simulink model "AESEncryption_21821"  (R2018b)
settings: Solver=FixedStepDiscrete  StartTime=0.0  StopTime=10  RelTol=1e-3
undefined symbols (not defined in the file or in its folder): gray
libraries: hdlsllib x5, visionsources x1, dspmtrx3 x1
settings Model: Creator=Administrator  LastModifiedBy=Administrator
settings OptimizationCC: BlockReduction=off  ConditionallyExecuteInputs=off  DefaultParameterBehavior=Inlined
settings DebuggingCC: AlgebraicLoopMsg=error  SingleTaskRateTransMsg=error
settings HardwareCC: ProdBitPerPointer=32  ProdBitPerSizeT=32  ProdBitPerPtrDiffT=32  ProdLargestAtomicFloat=None  ProdIntDivRoundTo=Undefined  ProdEndianess=Unspecified  ProdWordSize=32  ProdHWDeviceType=ASIC/FPGA->ASIC/FPGA  TargetBitPerPointer=64  TargetBitPerSizeT=64  TargetBitPerPtrDiffT=64  TargetLongLongMode=on  TargetIntDivRoundTo=Zero  TargetEndianess=LittleEndian  TargetWordSize=64  TargetHWDeviceType=Custom Processor->MATLAB Host Computer  ProdEqTarget=off

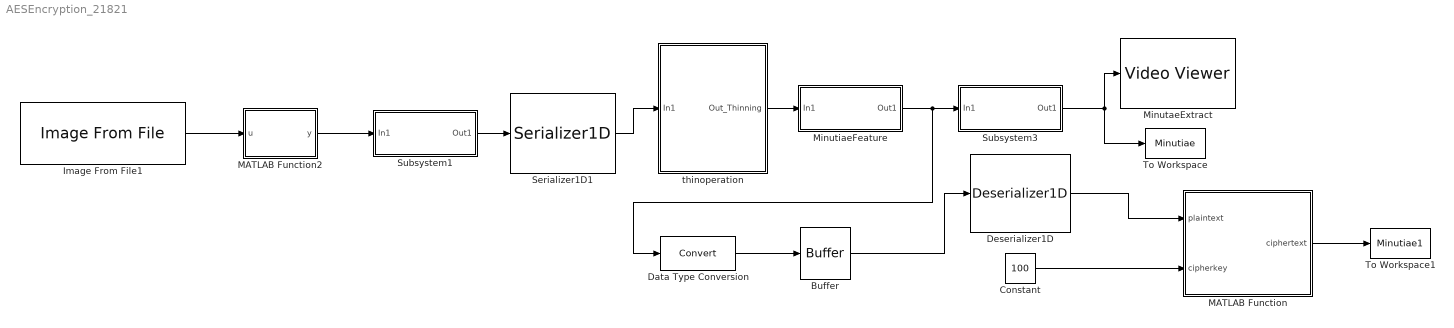
== system AESEncryption_21821 ==
  Buffer : Buffer  N=8192  OutputFrames=off
  Constant : Constant  Value=100  OutDataTypeStr=double
  Data Type Conversion : DataTypeConversion
  Deserializer1D : hdlsllib/HDL Operations/Deserializer1D  Ratio=128  IdleCycles=0  InitialCondition=0  startIn=off  validIn=off  validOut=off  inputDataDimensions=-1  inputSampleTime=-1  inputSignalType=auto
      settings: SourceProductName=HDL Coder  SourceProductBaseCode=HD
  Image From File1 : visionsources/Image From File  Tag=vipblks_nd  FileName=C:\Users\Administrator\Desktop\chapter\101_4.tif  imagePorts=One multidimensional signal  Ts=0.1  ImageDataType=uint8  Signed=on  WordLength=16  sdImageDataType=uint(8)  FractionLengthMode=User-defined  FractionLength=15  OutPortLabels=R|G|B
      settings: SourceProductName=Computer Vision System Toolbox
  MATLAB Function : MATLAB Function  TreatAsAtomicUnit=on
  MATLAB Function2 : MATLAB Function  TreatAsAtomicUnit=on
  MinutaeExtract : VideoViewer  colormapValue=gray(256)  FigPos=[367 903 376 593]
  MinutiaeFeature : Subsystem  TreatAsAtomicUnit=on
  Serializer1D1 : hdlsllib/HDL Operations/Serializer1D  Ratio=1  IdleCycles=0  validIn=off  startOut=off  validOut=off  inputDataDimensions=8192  inputSampleTime=-1  inputSignalType=auto
      settings: SourceProductName=HDL Coder  SourceProductBaseCode=HD
  Subsystem1 : Subsystem
  Subsystem3 : Subsystem
  To Workspace : ToWorkspace  VariableName=Minutiae  SampleTime=-1
      settings: Save2DSignal=2-D array (concatenate along first dimension)
  To Workspace1 : ToWorkspace  VariableName=Minutiae1  SampleTime=-1
      settings: Save2DSignal=2-D array (concatenate along first dimension)
  thinoperation : Subsystem  TreatAsAtomicUnit=on
  wires:
  Serializer1D1/1 -> thinoperation/1(In1)
  MATLAB Function2/1(y) -> Subsystem1/1(In1)
  Image From File1/1 -> MATLAB Function2/1(u)
  Subsystem1/1(Out1) -> Serializer1D1/1
  thinoperation/1(Out_Thinning) -> MinutiaeFeature/1(In1)
  Subsystem3/1(Out1) -> MinutaeExtract/1, To Workspace/1
  MATLAB Function/1(ciphertext) -> To Workspace1/1
  Constant/1 -> MATLAB Function/2(cipherkey)
  Deserializer1D/1 -> MATLAB Function/1(plaintext)
  MinutiaeFeature/1(Out1) -> Data Type Conversion/1, Subsystem3/1(In1)
  Data Type Conversion/1 -> Buffer/1
  Buffer/1 -> Deserializer1D/1

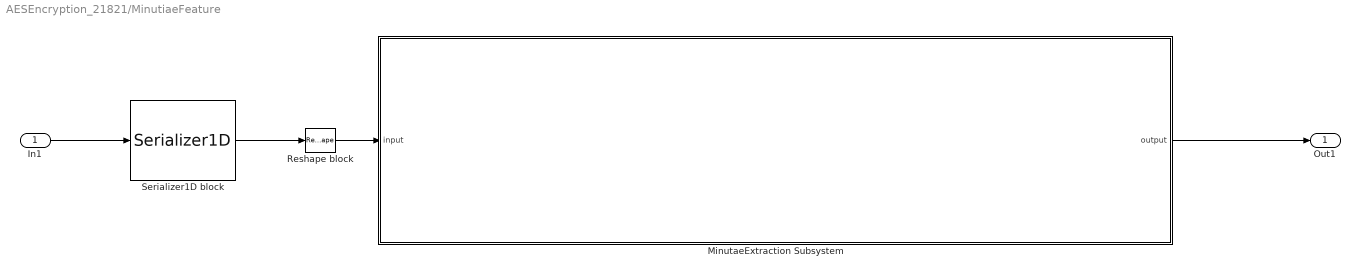
== system AESEncryption_21821/MinutiaeFeature ==
  In1 : Inport
  MinutaeExtraction Subsystem : Subsystem  TreatAsAtomicUnit=on
  Reshape block : Reshape  OutputDimensionality=Customize  OutputDimensions=[128,64]
  Serializer1D block : hdlsllib/HDL Operations/Serializer1D  Ratio=1  IdleCycles=0  validIn=off  startOut=off  validOut=off  inputDataDimensions=8192  inputSampleTime=-1  inputSignalType=auto
      settings: SourceProductName=HDL Coder  SourceProductBaseCode=HD
  Out1 : Outport
  wires:
  In1/1 -> Serializer1D block/1
  MinutaeExtraction Subsystem/1(output) -> Out1/1
  Reshape block/1 -> MinutaeExtraction Subsystem/1(input)
  Serializer1D block/1 -> Reshape block/1

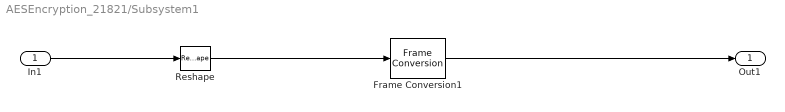
== system AESEncryption_21821/Subsystem1 ==
  In1 : Inport
  Frame Conversion1 : FrameConversion  OutFrame=Sample-based
  Reshape : Reshape
  Out1 : Outport
  wires:
  Frame Conversion1/1 -> Out1/1
  Reshape/1 -> Frame Conversion1/1
  In1/1 -> Reshape/1

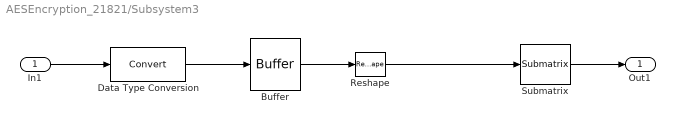
== system AESEncryption_21821/Subsystem3 ==
  In1 : Inport
  Buffer : Buffer  N=8192  OutputFrames=off
  Data Type Conversion : DataTypeConversion
  Reshape : Reshape  OutputDimensionality=Customize  OutputDimensions=[128,64]
  Submatrix : dspmtrx3/Submatrix  RowSpan=Range of rows  RowStartMode=First  RowStartIndex=1  RowEndMode=Last  RowEndIndex=1  ColSpan=Range of columns  ColStartMode=First  ColStartIndex=1  ColEndMode=Last  ColEndIndex=1
  Out1 : Outport
  wires:
  Data Type Conversion/1 -> Buffer/1
  Buffer/1 -> Reshape/1
  Reshape/1 -> Submatrix/1
  Submatrix/1 -> Out1/1
  In1/1 -> Data Type Conversion/1

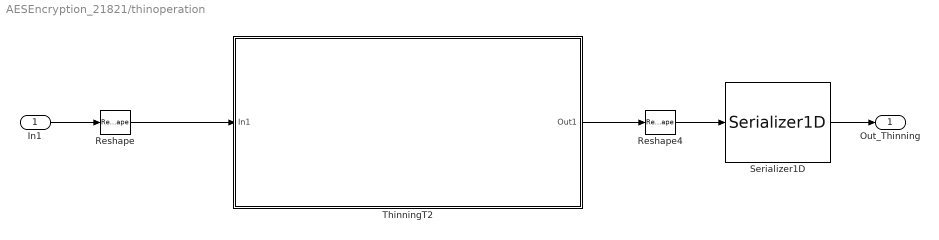
== system AESEncryption_21821/thinoperation ==
  In1 : Inport
  Reshape : Reshape  OutputDimensionality=Customize  OutputDimensions=[128,64]
  Reshape4 : Reshape  OutputDimensionality=Column vector (2-D)  OutputDimensions=[128,64]
  Serializer1D : hdlsllib/HDL Operations/Serializer1D  Ratio=1  IdleCycles=0  validIn=off  startOut=off  validOut=off  inputDataDimensions=-1  inputSampleTime=-1  inputSignalType=auto
      settings: SourceProductName=HDL Coder  SourceProductBaseCode=HD
  ThinningT2 : Subsystem  TreatAsAtomicUnit=on
  Out_Thinning : Outport
  wires:
  ThinningT2/1(Out1) -> Reshape4/1
  Reshape/1 -> ThinningT2/1(In1)
  Serializer1D/1 -> Out_Thinning/1
  In1/1 -> Reshape/1
  Reshape4/1 -> Serializer1D/1

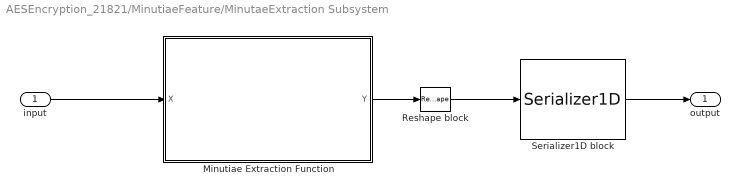
== system AESEncryption_21821/MinutiaeFeature/MinutaeExtraction Subsystem ==
  input : Inport
  Minutiae Extraction Function : MATLAB Function  TreatAsAtomicUnit=on
  Reshape block : Reshape  OutputDimensionality=Column vector (2-D)  OutputDimensions=[128,64]
  Serializer1D block : hdlsllib/HDL Operations/Serializer1D  Ratio=8192  IdleCycles=0  validIn=off  startOut=off  validOut=off  inputDataDimensions=-1  inputSampleTime=-1  inputSignalType=auto
      settings: SourceProductName=HDL Coder  SourceProductBaseCode=HD
  output : Outport
  wires:
  input/1 -> Minutiae Extraction Function/1(X)
  Serializer1D block/1 -> output/1
  Minutiae Extraction Function/1(Y) -> Reshape block/1
  Reshape block/1 -> Serializer1D block/1

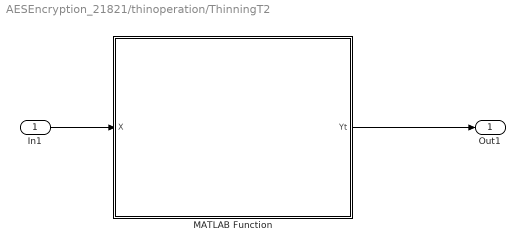
== system AESEncryption_21821/thinoperation/ThinningT2 ==
  In1 : Inport
  MATLAB Function : MATLAB Function  TreatAsAtomicUnit=on
  Out1 : Outport
  wires:
  In1/1 -> MATLAB Function/1(X)
  MATLAB Function/1(Yt) -> Out1/1

== matlab function AESEncryption_21821/MATLAB Function2 ==
  data: u input; y output
function y = fcn(u)
%#codegen
%i = rgb2gray(u);
b = u(100:227,150:213);
y = imbinarize(b);
%y = y(100:227,150:213);
%y = imbinarize(r);

== matlab function AESEncryption_21821/thinoperation/ThinningT2/MATLAB Function ==
  data: X input; Yt output
function Yt=thinningTh(X)
%img = imread ('2_4.jpg'); 
%Xr = rgb2gray(img);
%%%X = imbinarize(Xr);
%X = X(1:128,1:64);
[M,N]=size(X);
Yt = false(M,N);
Y=false(M,N,20);
Z=false(M,N,20);
Y(:,:,1)=X;
Z(:,:,1)=X;
for k=2:20
    Y(:,:,k)=Y(:,:,k-1);
    for i=2:M-1
        for j=2:N-1
            y11=Y(i-1,j-1,k);
            y12=Y(i-1,j,k);
            y13=Y(i-1,j+1,k);
            y21=Y(i,j-1,k);
            y22=Y(i,j,k);
            y23=Y(i,j+1,k);
            y31=Y(i+1,j-1,k);
            y32=Y(i+1,j,k);
            y33=Y(i+1,j+1,k);
            if y22==0
                if y11==1&&y12==1&&y13==1&&y31==0&&y32==0&&y33==0
                    Y(i,j,k)=1;
                elseif y11==1&&y13==0&&y21==1&&y23==0&&y31==1&&y33==0
                    Y(i,j,k)=1;
                elseif y11==0&&y12==0&&y13==0&&y31==1&&y32==1&&y33==1
                    Y(i,j,k)=1;
                elseif y11==0&&y13==1&&y21==0&&y23==1&&y31==0&&y33==1
                    Y(i,j,k)=1;
                elseif y12==1&&y13==1&&y21==0&&y23==1&&y32==0
                    Y(i,j,k)=1;
                elseif y11==1&&y12==1&&y21==1&&y23==0&&y32==0
                    Y(i,j,k)=1;
                elseif y12==0&&y21==1&&y23==0&&y31==1&&y21==1
                    Y(i,j,k)=1;
                elseif y12==0&&y21==0&&y23==1&&y32==1&&y33==1
                    Y(i,j,k)=1;
                    %extra
                elseif y11==0&&y12==0&&y23==1&&y31==1&&y32==1&&y33==1
                    Y(i,j,k)=1;
                end
            else
            end
        end
    end
%    Y(:,:,k)= Y(:,:,k-1);
     if Y(:,:,k)==Y(:,:,k-1)
%         break;
     end
end
Yt=Y(:,:,k);
%figure;
%imshow(Y);

== matlab function AESEncryption_21821/MATLAB Function ==
  data: plaintext input; ciphertext output; cipherkey input
%%%%%%%%%%%%%%%%%%%%%%%%%%%%%%%%%%%%%%%%%%%%%%%%%%%%%%%%%%%%%%%%%%%%%%%%%%
% MATLAB design: Advanced Encryption System (AES-128)
% [1] Advanced Encryption Standard (AES) (FIPS PUB 197)
%
% Key Design pattern covered in this example: 
% (1) This example uses fixed point and integer operators. 
% (2) Bitwise Operator support
%
%
% Note: This design is already in fixed point and suitable for HDL code
% generation. It is not advisable to run floating point to fixed point
% advisor on this design
%%%%%%%%%%%%%%%%%%%%%%%%%%%%%%%%%%%%%%%%%%%%%%%%%%%%%%%%%%%%%%%%%%%%%%%%%%

%   Copyright 2011-2015 The MathWorks, Inc.

%#codegen

%%%%%%%%%%%%%%%%%%%%%%%%%%%%%%%%%%%%%%%%%%%%%%%%%%%
% AES-128 Encryption
%
% plaintext:  text to be encrypted
% cipherkey:  key to encrypt plain text
% ciphertext: encrypted text
%%%%%%%%%%%%%%%%%%%%%%%%%%%%%%%%%%%%%%%%%%%%%%%%%%%
function ciphertext = mlhdlc_aes(plaintext, cipherkey)

    BS = 4;
    RS = 10;
    s = uint8(zeros(BS*BS, RS));
    k = uint8(zeros(BS*BS, RS));

    %%%%%%%%%%%%%%%%%%%%%%%%%%%%%%%%%%%%%%%%%%%%%%%%%%%
    % First round
    %%%%%%%%%%%%%%%%%%%%%%%%%%%%%%%%%%%%%%%%%%%%%%%%%%%
    s(:,1) = bitxor(plaintext, cipherkey);
    k(:,1) = ExtendKeys(cipherkey, 1);

    %%%%%%%%%%%%%%%%%%%%%%%%%%%%%%%%%%%%%%%%%%%%%%%%%%%
    % Second to tenth round
    %%%%%%%%%%%%%%%%%%%%%%%%%%%%%%%%%%%%%%%%%%%%%%%%%%%
    for i = 1:RS-1
        s(:, i+1) = mainroundstate(s(:, i), k(:, i));
        k(:, i+1) = ExtendKeys(k(:, i), i+1);
    end

    %%%%%%%%%%%%%%%%%%%%%%%%%%%%%%%%%%%%%%%%%%%%%%%%%%%
    % Final round
    %%%%%%%%%%%%%%%%%%%%%%%%%%%%%%%%%%%%%%%%%%%%%%%%%%%
    ciphertext = finalround(s(:, RS), k(:, RS));
end

%%%%%%%%%%%%%%%%%%%%%%%%%%%%%%%%%%%%%%%%%%%%%%%%%%%
% Main round state containing four steps:
% 1. SubBytes
% 2. ShiftRows
% 3. MixColumns
% 4. Xor text with key
%
% s_in:  text state from the previous round
% k_in:  initial key for the first round or 
%        extended round key for the other rounds
% s_out: text state to the next round
%%%%%%%%%%%%%%%%%%%%%%%%%%%%%%%%%%%%%%%%%%%%%%%%%%%
function s_out = mainroundstate(s_in, k_in)

    s1 = SubBytes(s_in);
    s2 = ShiftRows(s1);
    s3 = MixColumns(s2);
    s_out = bitxor(s3, k_in);
end

%%%%%%%%%%%%%%%%%%%%%%%%%%%%%%%%%%%%%%%%%%%%%%%%%%%
% Final round state containing only three steps:
% 1. SubBytes
% 2. ShiftRows
% 3. Xor text with key
%
% s_in:  text state from the previous round
% k_in:  extended round key for the last round
% s_out: the final cipher text
%%%%%%%%%%%%%%%%%%%%%%%%%%%%%%%%%%%%%%%%%%%%%%%%%%%
function s_out = finalround(s_in, k_in)

    s1 = SubBytes(s_in);
    s2 = ShiftRows(s1);
    s_out = bitxor(s2, k_in);
end

%%%%%%%%%%%%%%%%%%%%%%%%%%%%%%%%%%%%%%%%%%%%%%%%%%%%%%%%%%%%%%%%%%%%%%%%%%%
% Key extension
% Given initial key or the round key from the previous round via k_in and
% the round number as iter, outputs the key for the current round.
% For example, to calculate the round key for round 1, k_in is the initial
% key and iter is 1.
%
% k_in:  key from the previous round
% iter:  the round number, ranging from 1 to 10
% k_out: extended round key
%%%%%%%%%%%%%%%%%%%%%%%%%%%%%%%%%%%%%%%%%%%%%%%%%%%%%%%%%%%%%%%%%%%%%%%%%%%
function k_out = ExtendKeys(k_in, iter)

BS = 4;
sbox = [ ...
	hex2dec('63'), hex2dec('7c'), hex2dec('77'), hex2dec('7b'), hex2dec('f2'), hex2dec('6b'), hex2dec('6f'), hex2dec('c5'), hex2dec('30'), hex2dec('01'), hex2dec('67'), hex2dec('2b'), hex2dec('fe'), hex2dec('d7'), hex2dec('ab'), hex2dec('76'), ... %0
	hex2dec('ca'), hex2dec('82'), hex2dec('c9'), hex2dec('7d'), hex2dec('fa'), hex2dec('59'), hex2dec('47'), hex2dec('f0'), hex2dec('ad'), hex2dec('d4'), hex2dec('a2'), hex2dec('af'), hex2dec('9c'), hex2dec('a4'), hex2dec('72'), hex2dec('c0'), ... %1
	hex2dec('b7'), hex2dec('fd'), hex2dec('93'), hex2dec('26'), hex2dec('36'), hex2dec('3f'), hex2dec('f7'), hex2dec('cc'), hex2dec('34'), hex2dec('a5'), hex2dec('e5'), hex2dec('f1'), hex2dec('71'), hex2dec('d8'), hex2dec('31'), hex2dec('15'), ... %2
	hex2dec('04'), hex2dec('c7'), hex2dec('23'), hex2dec('c3'), hex2dec('18'), hex2dec('96'), hex2dec('05'), hex2dec('9a'), hex2dec('07'), hex2dec('12'), hex2dec('80'), hex2dec('e2'), hex2dec('eb'), hex2dec('27'), hex2dec('b2'), hex2dec('75'), ... %3
	hex2dec('09'), hex2dec('83'), hex2dec('2c'), hex2dec('1a'), hex2dec('1b'), hex2dec('6e'), hex2dec('5a'), hex2dec('a0'), hex2dec('52'), hex2dec('3b'), hex2dec('d6'), hex2dec('b3'), hex2dec('29'), hex2dec('e3'), hex2dec('2f'), hex2dec('84'), ... %4
	hex2dec('53'), hex2dec('d1'), hex2dec('00'), hex2dec('ed'), hex2dec('20'), hex2dec('fc'), hex2dec('b1'), hex2dec('5b'), hex2dec('6a'), hex2dec('cb'), hex2dec('be'), hex2dec('39'), hex2dec('4a'), hex2dec('4c'), hex2dec('58'), hex2dec('cf'), ... %5
	hex2dec('d0'), hex2dec('ef'), hex2dec('aa'), hex2dec('fb'), hex2dec('43'), hex2dec('4d'), hex2dec('33'), hex2dec('85'), hex2dec('45'), hex2dec('f9'), hex2dec('02'), hex2dec('7f'), hex2dec('50'), hex2dec('3c'), hex2dec('9f'), hex2dec('a8'), ... %6
	hex2dec('51'), hex2dec('a3'), hex2dec('40'), hex2dec('8f'), hex2dec('92'), hex2dec('9d'), hex2dec('38'), hex2dec('f5'), hex2dec('bc'), hex2dec('b6'), hex2dec('da'), hex2dec('21'), hex2dec('10'), hex2dec('ff'), hex2dec('f3'), hex2dec('d2'), ... %7
	hex2dec('cd'), hex2dec('0c'), hex2dec('13'), hex2dec('ec'), hex2dec('5f'), hex2dec('97'), hex2dec('44'), hex2dec('17'), hex2dec('c4'), hex2dec('a7'), hex2dec('7e'), hex2dec('3d'), hex2dec('64'), hex2dec('5d'), hex2dec('19'), hex2dec('73'), ... %8
	hex2dec('60'), hex2dec('81'), hex2dec('4f'), hex2dec('dc'), hex2dec('22'), hex2dec('2a'), hex2dec('90'), hex2dec('88'), hex2dec('46'), hex2dec('ee'), hex2dec('b8'), hex2dec('14'), hex2dec('de'), hex2dec('5e'), hex2dec('0b'), hex2dec('db'), ... %9
	hex2dec('e0'), hex2dec('32'), hex2dec('3a'), hex2dec('0a'), hex2dec('49'), hex2dec('06'), hex2dec('24'), hex2dec('5c'), hex2dec('c2'), hex2dec('d3'), hex2dec('ac'), hex2dec('62'), hex2dec('91'), hex2dec('95'), hex2dec('e4'), hex2dec('79'), ... %A
	hex2dec('e7'), hex2dec('c8'), hex2dec('37'), hex2dec('6d'), hex2dec('8d'), hex2dec('d5'), hex2dec('4e'), hex2dec('a9'), hex2dec('6c'), hex2dec('56'), hex2dec('f4'), hex2dec('ea'), hex2dec('65'), hex2dec('7a'), hex2dec('ae'), hex2dec('08'), ... %B
	hex2dec('ba'), hex2dec('78'), hex2dec('25'), hex2dec('2e'), hex2dec('1c'), hex2dec('a6'), hex2dec('b4'), hex2dec('c6'), hex2dec('e8'), hex2dec('dd'), hex2dec('74'), hex2dec('1f'), hex2dec('4b'), hex2dec('bd'), hex2dec('8b'), hex2dec('8a'), ... %C
	hex2dec('70'), hex2dec('3e'), hex2dec('b5'), hex2dec('66'), hex2dec('48'), hex2dec('03'), hex2dec('f6'), hex2dec('0e'), hex2dec('61'), hex2dec('35'), hex2dec('57'), hex2dec('b9'), hex2dec('86'), hex2dec('c1'), hex2dec('1d'), hex2dec('9e'), ... %D
	hex2dec('e1'), hex2dec('f8'), hex2dec('98'), hex2dec('11'), hex2dec('69'), hex2dec('d9'), hex2dec('8e'), hex2dec('94'), hex2dec('9b'), hex2dec('1e'), hex2dec('87'), hex2dec('e9'), hex2dec('ce'), hex2dec('55'), hex2dec('28'), hex2dec('df'), ... %E
	hex2dec('8c'), hex2dec('a1'), hex2dec('89'), hex2dec('0d'), hex2dec('bf'), hex2dec('e6'), hex2dec('42'), hex2dec('68'), hex2dec('41'), hex2dec('99'), hex2dec('2d'), hex2dec('0f'), hex2dec('b0'), hex2dec('54'), hex2dec('bb'), hex2dec('16')  ... %F
];

Rcon= uint8([ ...
	hex2dec('8d'), hex2dec('01'), hex2dec('02'), hex2dec('04'), hex2dec('08'), hex2dec('10'), hex2dec('20'), hex2dec('40'), hex2dec('80'), hex2dec('1b'), hex2dec('36'), hex2dec('6c'), hex2dec('d8'), hex2dec('ab'), hex2dec('4d'), hex2dec('9a'), ...
	hex2dec('2f'), hex2dec('5e'), hex2dec('bc'), hex2dec('63'), hex2dec('c6'), hex2dec('97'), hex2dec('35'), hex2dec('6a'), hex2dec('d4'), hex2dec('b3'), hex2dec('7d'), hex2dec('fa'), hex2dec('ef'), hex2dec('c5'), hex2dec('91'), hex2dec('39'), ...
	hex2dec('72'), hex2dec('e4'), hex2dec('d3'), hex2dec('bd'), hex2dec('61'), hex2dec('c2'), hex2dec('9f'), hex2dec('25'), hex2dec('4a'), hex2dec('94'), hex2dec('33'), hex2dec('66'), hex2dec('cc'), hex2dec('83'), hex2dec('1d'), hex2dec('3a'), ...
	hex2dec('74'), hex2dec('e8'), hex2dec('cb'), hex2dec('8d'), hex2dec('01'), hex2dec('02'), hex2dec('04'), hex2dec('08'), hex2dec('10'), hex2dec('20'), hex2dec('40'), hex2dec('80'), hex2dec('1b'), hex2dec('36'), hex2dec('6c'), hex2dec('d8'), ...
	hex2dec('ab'), hex2dec('4d'), hex2dec('9a'), hex2dec('2f'), hex2dec('5e'), hex2dec('bc'), hex2dec('63'), hex2dec('c6'), hex2dec('97'), hex2dec('35'), hex2dec('6a'), hex2dec('d4'), hex2dec('b3'), hex2dec('7d'), hex2dec('fa'), hex2dec('ef'), ...
	hex2dec('c5'), hex2dec('91'), hex2dec('39'), hex2dec('72'), hex2dec('e4'), hex2dec('d3'), hex2dec('bd'), hex2dec('61'), hex2dec('c2'), hex2dec('9f'), hex2dec('25'), hex2dec('4a'), hex2dec('94'), hex2dec('33'), hex2dec('66'), hex2dec('cc'), ...
	hex2dec('83'), hex2dec('1d'), hex2dec('3a'), hex2dec('74'), hex2dec('e8'), hex2dec('cb'), hex2dec('8d'), hex2dec('01'), hex2dec('02'), hex2dec('04'), hex2dec('08'), hex2dec('10'), hex2dec('20'), hex2dec('40'), hex2dec('80'), hex2dec('1b'), ...
	hex2dec('36'), hex2dec('6c'), hex2dec('d8'), hex2dec('ab'), hex2dec('4d'), hex2dec('9a'), hex2dec('2f'), hex2dec('5e'), hex2dec('bc'), hex2dec('63'), hex2dec('c6'), hex2dec('97'), hex2dec('35'), hex2dec('6a'), hex2dec('d4'), hex2dec('b3'), ...
	hex2dec('7d'), hex2dec('fa'), hex2dec('ef'), hex2dec('c5'), hex2dec('91'), hex2dec('39'), hex2dec('72'), hex2dec('e4'), hex2dec('d3'), hex2dec('bd'), hex2dec('61'), hex2dec('c2'), hex2dec('9f'), hex2dec('25'), hex2dec('4a'), hex2dec('94'), ...
	hex2dec('33'), hex2dec('66'), hex2dec('cc'), hex2dec('83'), hex2dec('1d'), hex2dec('3a'), hex2dec('74'), hex2dec('e8'), hex2dec('cb'), hex2dec('8d'), hex2dec('01'), hex2dec('02'), hex2dec('04'), hex2dec('08'), hex2dec('10'), hex2dec('20'), ...
	hex2dec('40'), hex2dec('80'), hex2dec('1b'), hex2dec('36'), hex2dec('6c'), hex2dec('d8'), hex2dec('ab'), hex2dec('4d'), hex2dec('9a'), hex2dec('2f'), hex2dec('5e'), hex2dec('bc'), hex2dec('63'), hex2dec('c6'), hex2dec('97'), hex2dec('35'), ...
	hex2dec('6a'), hex2dec('d4'), hex2dec('b3'), hex2dec('7d'), hex2dec('fa'), hex2dec('ef'), hex2dec('c5'), hex2dec('91'), hex2dec('39'), hex2dec('72'), hex2dec('e4'), hex2dec('d3'), hex2dec('bd'), hex2dec('61'), hex2dec('c2'), hex2dec('9f'), ...
	hex2dec('25'), hex2dec('4a'), hex2dec('94'), hex2dec('33'), hex2dec('66'), hex2dec('cc'), hex2dec('83'), hex2dec('1d'), hex2dec('3a'), hex2dec('74'), hex2dec('e8'), hex2dec('cb'), hex2dec('8d'), hex2dec('01'), hex2dec('02'), hex2dec('04'), ...
	hex2dec('08'), hex2dec('10'), hex2dec('20'), hex2dec('40'), hex2dec('80'), hex2dec('1b'), hex2dec('36'), hex2dec('6c'), hex2dec('d8'), hex2dec('ab'), hex2dec('4d'), hex2dec('9a'), hex2dec('2f'), hex2dec('5e'), hex2dec('bc'), hex2dec('63'), ...
	hex2dec('c6'), hex2dec('97'), hex2dec('35'), hex2dec('6a'), hex2dec('d4'), hex2dec('b3'), hex2dec('7d'), hex2dec('fa'), hex2dec('ef'), hex2dec('c5'), hex2dec('91'), hex2dec('39'), hex2dec('72'), hex2dec('e4'), hex2dec('d3'), hex2dec('bd'), ...
	hex2dec('61'), hex2dec('c2'), hex2dec('9f'), hex2dec('25'), hex2dec('4a'), hex2dec('94'), hex2dec('33'), hex2dec('66'), hex2dec('cc'), hex2dec('83'), hex2dec('1d'), hex2dec('3a'), hex2dec('74'), hex2dec('e8'), hex2dec('cb') ...
]);


k_out = uint8(zeros(BS*BS, 1));

% Pick the last column and rotate down by 1 (i.e. RotWord)
k_temp = [k_in((2-1)*BS + BS), k_in((3-1)*BS + BS), k_in((4-1)*BS + BS), k_in((1-1)*BS + BS)];
% Substitute RotWord with SBox
idx = k_temp + 1;
k_temp1 = sbox(uint8(idx));
% Xor the substituted RotWord with Rcon(iter)
k_temp2 = [bitxor(k_temp1(1), Rcon(uint8(iter + 1))), k_temp1(2:BS)];

% Calculate the first column of the new round key 
k_out((1-1)*BS + 1) = bitxor(k_in((1-1)*BS + 1), k_temp2(1));
k_out((2-1)*BS + 1) = bitxor(k_in((2-1)*BS + 1), k_temp2(2));
k_out((3-1)*BS + 1) = bitxor(k_in((3-1)*BS + 1), k_temp2(3));
k_out((4-1)*BS + 1) = bitxor(k_in((4-1)*BS + 1), k_temp2(4));

% Calculated the rest columns of the new round key
for i = 2:BS
    k_out((1-1)*BS + i) = bitxor(k_in((1-1)*BS + i), k_out((1-1)*BS + i - 1));
    k_out((2-1)*BS + i) = bitxor(k_in((2-1)*BS + i), k_out((2-1)*BS + i - 1));
    k_out((3-1)*BS + i) = bitxor(k_in((3-1)*BS + i), k_out((3-1)*BS + i - 1));
    k_out((4-1)*BS + i) = bitxor(k_in((4-1)*BS + i), k_out((4-1)*BS + i - 1));
end

end


%%%%%%%%%%%%%%%%%%%%%%%%%%%%%%%%%%%%%%%%%%%%%%%%%%%
% The SubBytes step
%%%%%%%%%%%%%%%%%%%%%%%%%%%%%%%%%%%%%%%%%%%%%%%%%%%
function s_out = SubBytes(s_in)

BS = 4;
sbox = [ ...
	hex2dec('63'), hex2dec('7c'), hex2dec('77'), hex2dec('7b'), hex2dec('f2'), hex2dec('6b'), hex2dec('6f'), hex2dec('c5'), hex2dec('30'), hex2dec('01'), hex2dec('67'), hex2dec('2b'), hex2dec('fe'), hex2dec('d7'), hex2dec('ab'), hex2dec('76'), ... %0
	hex2dec('ca'), hex2dec('82'), hex2dec('c9'), hex2dec('7d'), hex2dec('fa'), hex2dec('59'), hex2dec('47'), hex2dec('f0'), hex2dec('ad'), hex2dec('d4'), hex2dec('a2'), hex2dec('af'), hex2dec('9c'), hex2dec('a4'), hex2dec('72'), hex2dec('c0'), ... %1
	hex2dec('b7'), hex2dec('fd'), hex2dec('93'), hex2dec('26'), hex2dec('36'), hex2dec('3f'), hex2dec('f7'), hex2dec('cc'), hex2dec('34'), hex2dec('a5'), hex2dec('e5'), hex2dec('f1'), hex2dec('71'), hex2dec('d8'), hex2dec('31'), hex2dec('15'), ... %2
	hex2dec('04'), hex2dec('c7'), hex2dec('23'), hex2dec('c3'), hex2dec('18'), hex2dec('96'), hex2dec('05'), hex2dec('9a'), hex2dec('07'), hex2dec('12'), hex2dec('80'), hex2dec('e2'), hex2dec('eb'), hex2dec('27'), hex2dec('b2'), hex2dec('75'), ... %3
	hex2dec('09'), hex2dec('83'), hex2dec('2c'), hex2dec('1a'), hex2dec('1b'), hex2dec('6e'), hex2dec('5a'), hex2dec('a0'), hex2dec('52'), hex2dec('3b'), hex2dec('d6'), hex2dec('b3'), hex2dec('29'), hex2dec('e3'), hex2dec('2f'), hex2dec('84'), ... %4
	hex2dec('53'), hex2dec('d1'), hex2dec('00'), hex2dec('ed'), hex2dec('20'), hex2dec('fc'), hex2dec('b1'), hex2dec('5b'), hex2dec('6a'), hex2dec('cb'), hex2dec('be'), hex2dec('39'), hex2dec('4a'), hex2dec('4c'), hex2dec('58'), hex2dec('cf'), ... %5
	hex2dec('d0'), hex2dec('ef'), hex2dec('aa'), hex2dec('fb'), hex2dec('43'), hex2dec('4d'), hex2dec('33'), hex2dec('85'), hex2dec('45'), hex2dec('f9'), hex2dec('02'), hex2dec('7f'), hex2dec('50'), hex2dec('3c'), hex2dec('9f'), hex2dec('a8'), ... %6
	hex2dec('51'), hex2dec('a3'), hex2dec('40'), hex2dec('8f'), hex2dec('92'), hex2dec('9d'), hex2dec('38'), hex2dec('f5'), hex2dec('bc'), hex2dec('b6'), hex2dec('da'), hex2dec('21'), hex2dec('10'), hex2dec('ff'), hex2dec('f3'), hex2dec('d2'), ... %7
	hex2dec('cd'), hex2dec('0c'), hex2dec('13'), hex2dec('ec'), hex2dec('5f'), hex2dec('97'), hex2dec('44'), hex2dec('17'), hex2dec('c4'), hex2dec('a7'), hex2dec('7e'), hex2dec('3d'), hex2dec('64'), hex2dec('5d'), hex2dec('19'), hex2dec('73'), ... %8
	hex2dec('60'), hex2dec('81'), hex2dec('4f'), hex2dec('dc'), hex2dec('22'), hex2dec('2a'), hex2dec('90'), hex2dec('88'), hex2dec('46'), hex2dec('ee'), hex2dec('b8'), hex2dec('14'), hex2dec('de'), hex2dec('5e'), hex2dec('0b'), hex2dec('db'), ... %9
	hex2dec('e0'), hex2dec('32'), hex2dec('3a'), hex2dec('0a'), hex2dec('49'), hex2dec('06'), hex2dec('24'), hex2dec('5c'), hex2dec('c2'), hex2dec('d3'), hex2dec('ac'), hex2dec('62'), hex2dec('91'), hex2dec('95'), hex2dec('e4'), hex2dec('79'), ... %A
	hex2dec('e7'), hex2dec('c8'), hex2dec('37'), hex2dec('6d'), hex2dec('8d'), hex2dec('d5'), hex2dec('4e'), hex2dec('a9'), hex2dec('6c'), hex2dec('56'), hex2dec('f4'), hex2dec('ea'), hex2dec('65'), hex2dec('7a'), hex2dec('ae'), hex2dec('08'), ... %B
	hex2dec('ba'), hex2dec('78'), hex2dec('25'), hex2dec('2e'), hex2dec('1c'), hex2dec('a6'), hex2dec('b4'), hex2dec('c6'), hex2dec('e8'), hex2dec('dd'), hex2dec('74'), hex2dec('1f'), hex2dec('4b'), hex2dec('bd'), hex2dec('8b'), hex2dec('8a'), ... %C
	hex2dec('70'), hex2dec('3e'), hex2dec('b5'), hex2dec('66'), hex2dec('48'), hex2dec('03'), hex2dec('f6'), hex2dec('0e'), hex2dec('61'), hex2dec('35'), hex2dec('57'), hex2dec('b9'), hex2dec('86'), hex2dec('c1'), hex2dec('1d'), hex2dec('9e'), ... %D
	hex2dec('e1'), hex2dec('f8'), hex2dec('98'), hex2dec('11'), hex2dec('69'), hex2dec('d9'), hex2dec('8e'), hex2dec('94'), hex2dec('9b'), hex2dec('1e'), hex2dec('87'), hex2dec('e9'), hex2dec('ce'), hex2dec('55'), hex2dec('28'), hex2dec('df'), ... %E
	hex2dec('8c'), hex2dec('a1'), hex2dec('89'), hex2dec('0d'), hex2dec('bf'), hex2dec('e6'), hex2dec('42'), hex2dec('68'), hex2dec('41'), hex2dec('99'), hex2dec('2d'), hex2dec('0f'), hex2dec('b0'), hex2dec('54'), hex2dec('bb'), hex2dec('16')  ... %F
];

s_out = fi(zeros(BS*BS, 1), 0, 8, 0);

for i=1:BS
    for j=1:BS
        idx = uint16(s_in((i-1)*BS + j)) + 1;
        s_out((i-1)*BS + j) = sbox(idx);
    end
end

end

%%%%%%%%%%%%%%%%%%%%%%%%%%%%%%%%%%%%%%%%%%%%%%%%%%%
% The ShiftRows step
%%%%%%%%%%%%%%%%%%%%%%%%%%%%%%%%%%%%%%%%%%%%%%%%%%%
function s_out = ShiftRows(s_in)

BS = 4;
s_out = uint8(zeros(BS*BS, 1));

s_out(1) = s_in(1); s_out(2) = s_in(2); s_out(3) = s_in(3); s_out(4) = s_in(4);
s_out(5) = s_in(6); s_out(6) = s_in(7); s_out(7) = s_in(8); s_out(8) = s_in(5);
s_out(9) = s_in(11); s_out(10) = s_in(12); s_out(11) = s_in(9); s_out(12) = s_in(10);
s_out(13) = s_in(16); s_out(14) = s_in(13); s_out(15) = s_in(14); s_out(16) = s_in(15);

end

%%%%%%%%%%%%%%%%%%%%%%%%%%%%%%%%%%%%%%%%%%%%%%%%%%%
% The MixColumns step
%%%%%%%%%%%%%%%%%%%%%%%%%%%%%%%%%%%%%%%%%%%%%%%%%%%
function s_out = MixColumns(s_in)

BS = 4;
s_out = uint8(zeros(BS*BS, 1));
e = uint8(zeros(BS, 1));

a = s_in;
b = bitsll(s_in, 1);
c = bitget(s_in, BS*2);
d = bitxor(b, c*hex2dec('1b')); % s_in * 2

for i = 1:BS
    e(i) = bitxor(bitxor(a((1-1)*BS + i), a((2-1)*BS + i)), bitxor(a((3-1)*BS + i), a((4-1)*BS + i)));
    s_out((1-1)*BS + i) = bitxor(bitxor(e(i), a((1-1)*BS + i)), bitxor(d((1-1)*BS + i), d((2-1)*BS + i)));
    s_out((2-1)*BS + i) = bitxor(bitxor(e(i), a((2-1)*BS + i)), bitxor(d((2-1)*BS + i), d((3-1)*BS + i)));
    s_out((3-1)*BS + i) = bitxor(bitxor(e(i), a((3-1)*BS + i)), bitxor(d((3-1)*BS + i), d((4-1)*BS + i)));
    s_out((4-1)*BS + i) = bitxor(bitxor(e(i), a((4-1)*BS + i)), bitxor(d((4-1)*BS + i), d((1-1)*BS + i)));
end

end

== matlab function AESEncryption_21821/MinutiaeFeature/MinutaeExtraction Subsystem/Minutiae Extraction Function ==
  data: X input; Y output
function Y=minuextractT(X)
%img = imread ('101_7.tif'); 
%Xr = rgb2gray(img);
%Xt = imbinarize(img);
%X=~bwmorph(Xt,'thin',Inf);
[M,N]=size(X);
%mi(:,:)=X;
Y=false(M,N);
Y(:,:)=X;
%[M,N]=size(X);
mi=false(M,N);

for i=2:M-1
    for j=2:N-1
        % * * * y11 y12 y13
        % * @ * y21 y22 y23
        % * * * y31 y32 y33
        y11=Y(i-1,j-1);
        y12=Y(i-1,j);
        y13=Y(i-1,j+1);
        y21=Y(i,j-1);
        y22=Y(i,j);
        y23=Y(i,j+1);
        y31=Y(i+1,j-1);
        y32=Y(i+1,j);
        y33=Y(i+1,j+1);
        if y22==0
            if y11+y12+y13+y23+y33+y31+y21+y32==7
                mi(i,j)=1;
            elseif y11==0 && y12==1 && y13==0 && y21==1 && y23==1 && y31==1 && y32==0 && y33==1
                mi(i,j)=2;
            elseif y11==1 && y12==0 && y13==1 && y21==1 && y23==1 && y31==0 && y32==1 && y33==0
                mi(i,j)=2;
            elseif y11==0 && y12==1 && y13==1 && y21==1 && y23==0 && y31==0 && y32==1 && y33==1
                mi(i,j)=2;
            elseif y11==1 && y12==1 && y13==0 && y21==0 && y23==1 && y31==1 && y32==1 && y33==0
                mi(i,j)=2;
            elseif y11==1 && y12==0 && y13==1 && y21==0 && y23==0 && y31==1 && y32==1 && y33==1
                mi(i,j)=2;
            elseif y11==1 && y12==1 && y13==1 && y21==0 && y23==0 && y31==1 && y32==0 && y33==1
                mi(i,j)=2;
            elseif y11==1 && y12==0 && y13==1 && y21==0 && y23==1 && y31==1 && y32==0 && y33==1
                mi(i,j)=2;
            elseif y11==1 && y12==0 && y13==1 && y21==1 && y23==0 && y31==1 && y32==0 && y33==1
                mi(i,j)=2;
            elseif y11==0 && y12==1 && y13==0 && y21==1 && y23==1 && y31==0 && y32==1 && y33==1
                mi(i,j)=2;
            elseif y11==0 && y12==1 && y13==1 && y21==1 && y23==1 && y31==0 && y32==1 && y33==0
                mi(i,j)=2;
            elseif y11==0 && y12==1 && y13==0 && y21==1 && y23==1 && y31==1 && y32==1 && y33==0
                mi(i,j)=2;
            elseif y11==1 && y12==1 && y13==0 && y21==1 && y23==1 && y31==0 && y32==1 && y33==0
                mi(i,j)=2;
            elseif y11==1 && y12==0 && y13==1 && y21==0 && y23==0 && y31==0 && y32==1 && y33==1
                mi(i,j)=2;
            elseif y11==1 && y12==0 && y13==1 && y21==0 && y23==0 && y31==1 && y32==1 && y33==0
                mi(i,j)=2;
            elseif y11==0 && y12==1 && y13==1 && y21==0 && y23==0 && y31==1 && y32==0 && y33==1
                mi(i,j)=2;
            elseif y11==1 && y12==1 && y13==0 && y21==0 && y23==0 && y31==1 && y32==0 && y33==1
                mi(i,j)=2;
            elseif y11==1 && y12==1 && y13==0 && y21==0 && y23==1 && y31==1 && y32==0 && y33==1
                mi(i,j)=2;
            elseif y11==1 && y12==0 && y13==1 && y21==1 && y23==0 && y31==0 && y32==1 && y33==1
                mi(i,j)=2;
            elseif y11==1 && y12==0 && y13==1 && y21==0 && y23==1 && y31==1 && y32==1 && y33==0
                mi(i,j)=2;
            elseif y11==0 && y12==1 && y13==1 && y21==1 && y23==0 && y31==1 && y32==0 && y33==1
                mi(i,j)=2;
            elseif y11==1 && y12==0 && y13==1 && y21==1 && y23==0 && y31==0 && y32==0 && y33==1
                mi(i,j)=2;
            elseif y11==0 && y12==0 && y13==1 && y21==1 && y23==0 && y31==1 && y32==0 && y33==1
                mi(i,j)=2;
            elseif y11==1 && y12==0 && y13==0 && y21==0 && y23==1 && y31==1 && y32==0 && y33==1
                mi(i,j)=2;
            elseif y11==1 && y12==0 && y13==1 && y21==0 && y23==1 && y31==1 && y32==0 && y33==0
                mi(i,j)=2;
            end
        else
        end
    end
end
 Y=mi(:,:);

% %false minutiae deletion
% for M=1:300
%     for N=1:200
%         if mi(M,N)==1||mi(M,N)==2
%             d=20;
%             if M<d||M+d>300||N<d||N+d>200
%                 mi(M,N)=0;
%             else
%             end
%         else
%         end
%     end
% end
% 
% for N=1:200
%     for M=1:300
%         if mi(M,N)==1||mi(M,N)==2
%             for i=1:300
%                 for j=1:200
%                     if mi(i,j)==1||mi(i,j)==2
%                         if mi(M,N)==mi(i,j)
%                             d=10;
%                         else
%                             d=5;
%                         end
%                         a=sqrt((M-i)^2+(N-j)^2);
%                         if a<d&&a>0
%                             mi(M,N)=0;
%                             mi(i,j)=0;
%                         else
%                         end
%                     end
%                 end
%             end
%         else
%         end
%     end
% end
% figure
% hold on
% for M=1:320
%     for N=1:240
%         if mi(M,N)==1
%             a=round((M-1)/12)+1;
%             b=round((N-1)/12)+1;
%             plot(1*(N++1i*(M)),'ro','LineWidth',2)
%         elseif mi(M,N)==2
%             a=round((M-1)/12)+1;
%             b=round((N-1)/12)+1;
%             plot(1*(N++1i*(M)),'bo','LineWidth',2)
%         end
%     end
% end

%figure;imshow(img);
%figure;imshow(Xr);
%figure;imshow(Xt);
%figure;imshow(X);
%figure;imshow(Y);
